simulink model "RP20231104WLR_231105"  (R2018b)
settings: Solver=FixedStepDiscrete  StartTime=0.0  StopTime=10.0  FixedStep=0.0005  RelTol=1e-3  EnableMultiTasking=on
undefined symbols (not defined in the file or in its folder): I_AN06_5V, I_AN07_5V, I_AN08_5V, I_AN09_5V, I_HALL1, I_SW01_L, O_SW12_HS1A, O_SW14_HS1A, PWM3
libraries: ec5744lib x60, simulink x33, canmsglib x5
(part 1 of 2)
settings Model: Creator=evil  LastModifiedBy=evil
settings SolverCC: AutoInsertRateTranBlk=on
settings OptimizationCC: DefaultParameterBehavior=Inlined  InlineInvariantSignals=on  EnhancedBackFolding=on  ExpressionFolding=off  PassReuseOutputArgsAs=Individual arguments  RollThreshold=65  StateBitsets=on  DataBitsets=on  ZeroExternalMemoryAtStartup=off  ZeroInternalMemoryAtStartup=off  EfficientFloat2IntCast=on  OptimizeBlockOrder=speed  DifferentSizesBufferReuse=on
settings DebuggingCC: InheritedTsInSrcMsg=none  ParameterTunabilityLossMsg=error
settings HardwareCC: ProdBitPerPointer=32  ProdBitPerSizeT=32  ProdBitPerPtrDiffT=32  ProdLargestAtomicInteger=Long  ProdLargestAtomicFloat=Double  ProdEndianess=BigEndian  ProdWordSize=32  ProdHWDeviceType=Freescale MPC5500
settings SFSimCC: MATLABDynamicMemAlloc=off
settings RTWCC: SystemTargetFile=ec5744.tlc  MakeCommand=make_rtw optimized_fixed_point=1  GenerateMakefile=off  TemplateMakefile=ec5744_lcc.tmf  PostCodeGenCommand=ec5744_pst_s2(buildInfo)  Description=Target for EC5744  GenerateReport=on  IncludeHyperlinkInReport=on  LaunchReport=on  GenerateTraceInfo=on  GenerateTraceReport=on  GenerateTraceReportSl=on  GenerateTraceReportSf=on  GenerateTraceReportEml=on
settings CodeAppCC: ForceParamTrailComments=on  IgnoreCustomStorageClasses=off  OperatorAnnotations=on  SimulinkDataObjDesc=on  SFDataObjDesc=on  InsertBlockDesc=on
settings STFCustomTargetCC: TargetLangStandard=C99 (ISO)  MultiwordLength=256  ModelReferenceCompliant=off  IncludeMdlTerminateFcn=off  CombineOutputUpdateFcns=on  SuppressErrorStatus=on  ERTCustomFileBanners=on  SupportContinuousTime=off  SupportNonInlinedSFcns=off  RemoveResetFunc=on  MATLABClassNameForMDSCustomization=Simulink.SoftwareTarget.ERTCustomization  SystemTargetFile=ec5744.tlc
settings ERTTargetCC: TargetLangStandard=C99 (ISO)  ModelReferenceCompliant=off  ParMdlRefBuildCompliant=off  CompOptLevelCompliant=off  ConcurrentExecutionCompliant=off  IncludeMdlTerminateFcn=off  SuppressErrorStatus=on  ModelStepFunctionPrototypeControlCompliant=off  CPPClassGenCompliant=off  UseToolchainInfoCompliant=off  GenerateASAP2=on  InlinedParameterPlacement=NonHierarchical  ERTSrcFileBannerTemplate=ec5744_code_template.cgt  ERTHdrFileBannerTemplate=ec5744_code_template.cgt  ERTDataSrcFileTemplate=ec5744_code_template.cgt  ERTDataHdrFileTemplate=ec5744_code_template.cgt  ERTCustomFileTemplate=ec5744_file_process.tlc

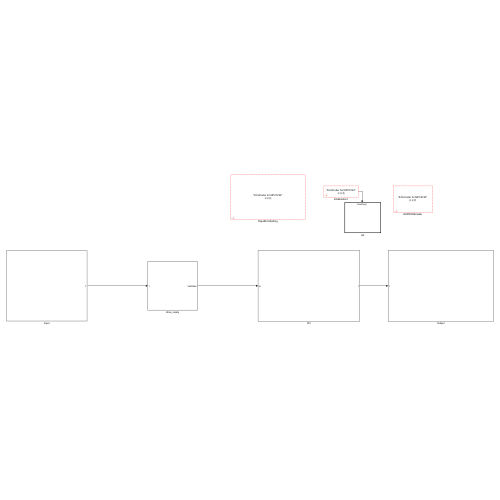
[thumbnail: Simulink's stored preview of the top-level diagram]
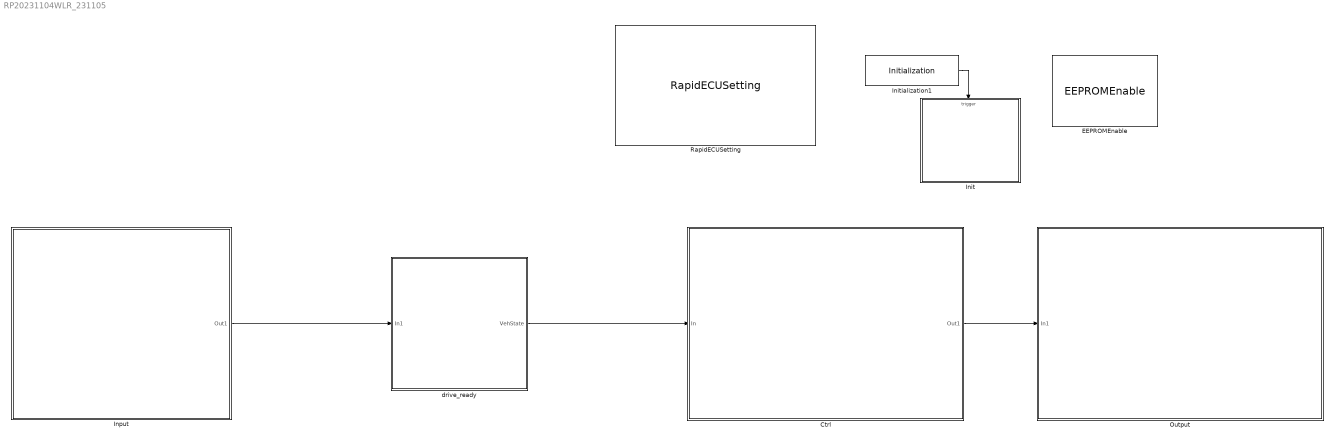
== system RP20231104WLR_231105 ==
  Ctrl : Subsystem
  EEPROMEnable : ec5744lib/RapidECU_U3/09MemoryManagement/EEPROMEnable  eepromenable=on
      settings: SourceProductName=ECUCoder for MPC5744
  Init : Subsystem  TreatAsAtomicUnit=on
  Initialization1 : ec5744lib/RapidECU_U3/08MCUManagement/Initialization
      settings: SourceProductName=ECUCoder for MPC5744
  Input : Subsystem
  Output : Subsystem
  RapidECUSetting : ec5744lib/RapidECU_U3/RapidECUSetting
      link override CAN: apdf=9  bpdf=4  cpdf=4  acmt=Extended(29-bit ID)  bcmt=Standard(11-bit ID)  ccmt=Standard(11-bit ID)
      link override LIN: abrt=19200
      settings: SourceProductName=ECUCoder for MPC5744
  drive_ready : Subsystem
  wires:
  Ctrl/1(Out1) -> Output/1(In1)
  Initialization1/1 -> Init/Trigger
  Input/1(Out1) -> drive_ready/1(In1)
  drive_ready/1(VehState) -> Ctrl/1(In)

== system RP20231104WLR_231105/Ctrl ==
  In : Inport
  10ms1 : simulink/Ports & Subsystems/Function-Call Generator  sample_time=0.01  numberOfIterations=1
  10ms5 : simulink/Ports & Subsystems/Function-Call Generator  sample_time=0.01  numberOfIterations=1
  Bus Creator1 : BusCreator  Inputs=3
  FAN_WP_CTRL : Subsystem  TreatAsAtomicUnit=on
  MoTrqReq : Subsystem  TreatAsAtomicUnit=on
  Out1 : Outport  VectorParamsAs1DForOutWhenUnconnected=on
  wires:
  10ms1/1 -> MoTrqReq/Trigger
  In/1 -> FAN_WP_CTRL/1(In), Bus Creator1/3, MoTrqReq/1(In)
  10ms5/1 -> FAN_WP_CTRL/Trigger
  MoTrqReq/1(Motor_CtrlBus) -> Bus Creator1/1  "Motor_CtrlBus"
  FAN_WP_CTRL/1(WP_FAN) -> Bus Creator1/2  "WP_FAN"
  Bus Creator1/1 -> Out1/1

== system RP20231104WLR_231105/Init ==
  function : TriggerPort  TriggerType=function-call  VariantControl=(inherit)
  AfterRunSwitch1 : ec5744lib/RapidECU_U3/05PowerManagement/AfterRunSwitch  sampletime=-1
      settings: SourceProductName=ECUCoder for MPC5744
  Constant : Constant  OutDataTypeStr=boolean
  Data Type Conversion : DataTypeConversion  OutDataTypeStr=boolean
  wires:
  Constant/1 -> Data Type Conversion/1
  Data Type Conversion/1 -> AfterRunSwitch1/1

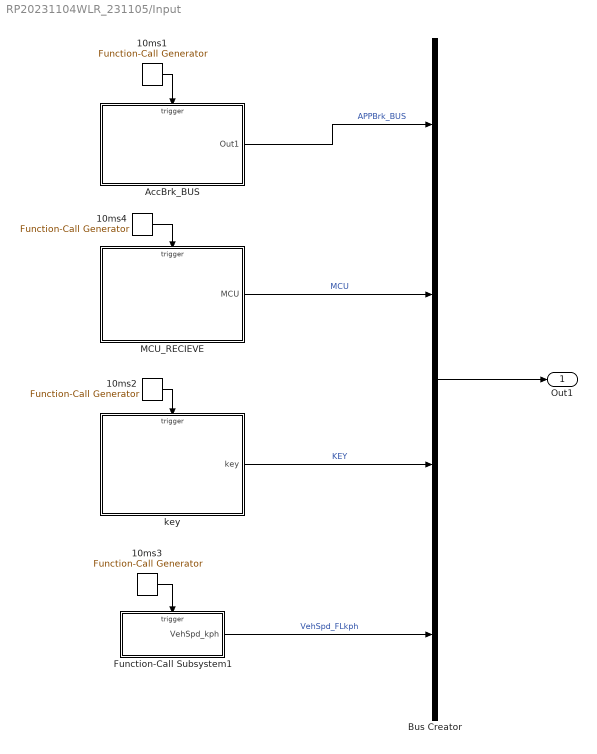
== system RP20231104WLR_231105/Input ==
  10ms{1..4} (4 alike) : simulink/Ports & Subsystems/Function-Call Generator  sample_time=0.01  numberOfIterations=1
  AccBrk_BUS : Subsystem  TreatAsAtomicUnit=on
  Bus Creator : BusCreator  Inputs=4
  Function-Call Subsystem1 : Subsystem  TreatAsAtomicUnit=on
  MCU_RECIEVE : Subsystem  TreatAsAtomicUnit=on
  key : Subsystem  TreatAsAtomicUnit=on
  Out1 : Outport  VectorParamsAs1DForOutWhenUnconnected=on
  wires:
  10ms1/1 -> AccBrk_BUS/Trigger
  MCU_RECIEVE/1(MCU) -> Bus Creator/2  "MCU"
  10ms4/1 -> MCU_RECIEVE/Trigger
  key/1(key) -> Bus Creator/3  "KEY"
  10ms2/1 -> key/Trigger
  Bus Creator/1 -> Out1/1
  AccBrk_BUS/1(Out1) -> Bus Creator/1  "APPBrk_BUS"
  10ms3/1 -> Function-Call Subsystem1/Trigger
  Function-Call Subsystem1/1(VehSpd_kph) -> Bus Creator/4  "VehSpd_FLkph"

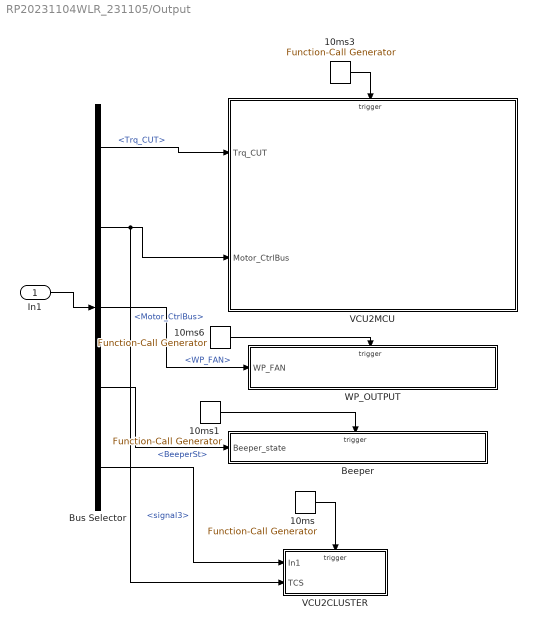
== system RP20231104WLR_231105/Output ==
  In1 : Inport
  10ms{,1,3,6} (4 alike) : simulink/Ports & Subsystems/Function-Call Generator  sample_time=0.01  numberOfIterations=1
  Beeper : Subsystem  TreatAsAtomicUnit=on
  Bus Selector : BusSelector  OutputSignals=signal3.signal2.APPBrk_BUS.Trq_CUT,Motor_CtrlBus,WP_FAN,signal3.VehState.BeeperSt,signal3
  VCU2CLUSTER : Subsystem  TreatAsAtomicUnit=on
  VCU2MCU : Subsystem  TreatAsAtomicUnit=on
  WP_OUTPUT : Subsystem  TreatAsAtomicUnit=on
  wires:
  10ms3/1 -> VCU2MCU/Trigger
  10ms6/1 -> WP_OUTPUT/Trigger
  In1/1 -> Bus Selector/1
  Bus Selector/1 -> VCU2MCU/1(Trq_CUT)  "<Trq_CUT>"
  Bus Selector/3 -> WP_OUTPUT/1(WP_FAN)  "<WP_FAN>"
  Bus Selector/2 -> VCU2CLUSTER/2(TCS), VCU2MCU/2(Motor_CtrlBus)  "<Motor_CtrlBus>"
  Bus Selector/4 -> Beeper/1(Beeper_state)  "<BeeperSt>"
  10ms1/1 -> Beeper/Trigger
  10ms/1 -> VCU2CLUSTER/Trigger
  Bus Selector/5 -> VCU2CLUSTER/1(In1)  "<signal3>"

== system RP20231104WLR_231105/drive_ready ==
  In1 : Inport
  10ms7 : simulink/Ports & Subsystems/Function-Call Generator  sample_time=0.01  numberOfIterations=1
  Bus Creator : BusCreator  Inputs=2
  Drive_ready : Subsystem  TreatAsAtomicUnit=on
  VehState : Outport
  wires:
  10ms7/1 -> Drive_ready/Trigger
  Drive_ready/1(VehStateBus) -> Bus Creator/1  "VehState"
  Bus Creator/1 -> VehState/1
  In1/1 -> Bus Creator/2, Drive_ready/1(BusIn)

== system RP20231104WLR_231105/Ctrl/FAN_WP_CTRL ==
  note: 1.温升做一个微分，根据温升速度来确定转速（温升系数）做到二维查表
      | 2.冷却要尽量做到刚刚好不过量，作热仿真（b站simulink热仿真）
  In : Inport
  function : TriggerPort  TriggerType=function-call  VariantControl=(inherit)
  Bus Creator : BusCreator  Inputs=1
  Bus Selector3 : BusSelector  OutputSignals=signal2.MCU.MCU_pwr.MCU_temp,signal2.MCU.MCU_pwr.motor_temp
  Data Type Conversion3 : DataTypeConversion  OutDataTypeStr=uint16
  Gain : Gain  Gain=10000/2000
  MCU__spd : Lookup_n-D  NumberOfTableDimensions=1  BreakpointsForDimension1=uint16([10,15,20,25,30,35,40,45,50,55,60,65,70,75]);  Table=uint16([0,0,600,600,600,600,800,800,800,1000,1000,1000,1000,1000]);  ExtrapMethod=Clip  InternalRulePriority=Speed  RndMeth=Simplest  InputSameDT=on
  MinMax : MinMax  Function=max  Inputs=2  OutDataTypeStr=uint16
  moter__spd : Lookup_n-D  NumberOfTableDimensions=1  BreakpointsForDimension1=uint16([0,10,20,30,40,50,60,70,80,90,100,110,120]);  Table=uint16([0,0,0,0,0,0,0,1400,1700,2000,2000,2000,2000]);  ExtrapMethod=Clip  InternalRulePriority=Speed  RndMeth=Simplest  InputSameDT=on
  WP_FAN : Outport  VectorParamsAs1DForOutWhenUnconnected=on
  wires:
  In/1 -> Bus Selector3/1
  Bus Selector3/1 -> MCU__spd/1  "<MCU_temp>"
  Bus Selector3/2 -> moter__spd/1  "<motor_temp>"
  MCU__spd/1 -> MinMax/1
  moter__spd/1 -> MinMax/2
  Bus Creator/1 -> WP_FAN/1
  MinMax/1 -> Gain/1  "Water_pump"
  Gain/1 -> Data Type Conversion3/1  "Water_pump"
  Data Type Conversion3/1 -> Bus Creator/1  "Water_pump"

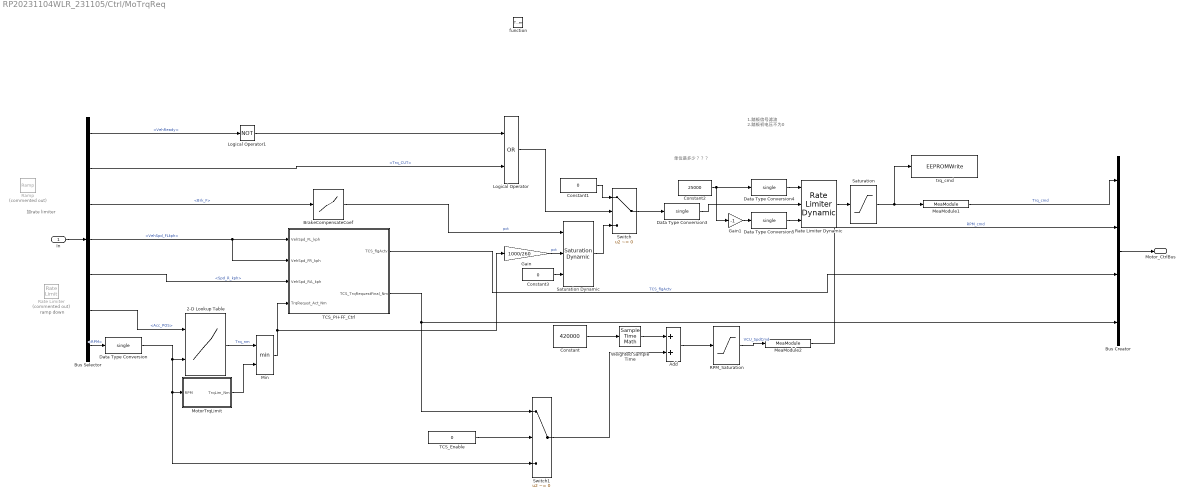
== system RP20231104WLR_231105/Ctrl/MoTrqReq ==
  note: 单位是多少？？？
  note: 加rate limiter
  note: ramp down
  note: 1.踏板信号滤波
      | 2.踏板初电压不为0
  In : Inport
  function : TriggerPort  TriggerType=function-call  VariantControl=(inherit)
  2-D Lookup Table : Lookup_n-D  BreakpointsForDimension1=single([0,10,20,30,40,50,60,70,80,90,100]);  BreakpointsForDimension2=single([200,400,600,800,1000,1200,1400,1600,1800,2000,2200,2400,2600,2800,3000,3500,4000,4500,5000,5200]);  BreakpointsForDimension1DataTypeStr=single  BreakpointsForDimension2DataTypeStr=single  Table=single(reshape([0,20,35,50,79,100,120,125,130,130,170,0,20,35,50,79,100,120,125,160,160,170,0,20,35,50,79,100,120,125,160,160,180,0,20,35,50,79,105,120,130,160,160,180,0,20,35,50,85,105,125,135,160,160,180,0,20,35,50,85,105,125,140,170,170,210,0,20,30,50,85,110,125,145,160,160,200,0,18,30,50,90,110,135,155,160,160,200,0,18,25,50,95,110,135,155,160,160,200,0,18,25,40,100,110,135,155,160,160,200,0,17,25,40,110,115,135,155,160,160,200,0,17,25,40,110,115,135,155,160,160,200,0,16,20,40,110,125,135,155,160,160,190,0,16,20,40,100,125,130,155,160,160,180,0,15,20,40,90,120,130,155,160,160,180,0,15,20,40,90,110,120,135,142,142,152,0,15,20,40,80,90,100,110,120,120,133,0,14,20,40,72,80,90,100,105,105,118,0,14,20,38,70,76,82,88,94,95,106,0,14,18,35,65,70,74,82,88,91,100],11,20));  InternalRulePriority=Speed  RndMeth=Simplest  InputSameDT=on
  Add : Sum
  BrakeCompensateCoef : Lookup_n-D  NumberOfTableDimensions=1  BreakpointsForDimension1=single([550,2000]);  Table=single([1000,0]);  ExtrapMethod=Clip  InternalRulePriority=Speed  OutDataTypeStr=single  RndMeth=Simplest  InputSameDT=on
  Bus Creator : BusCreator  Inputs=4
  Bus Selector : BusSelector  OutputSignals=VehState.VehReady,signal2.APPBrk_BUS.Trq_CUT,signal2.APPBrk_BUS.Brk_F,signal2.VehSpd_FLkph,signal2.MCU.MCU_state.Spd_R_kph,signal2.APPBrk_BUS.Acc_POS,signal2.MCU.MCU_state.RPM
  Constant : Constant  Value=420000  OutDataTypeStr=single
  Constant1 : Constant  Value=0  OutDataTypeStr=single
  Constant2 : Constant  Value=25000  OutDataTypeStr=single
  Constant3 : Constant  Value=0  OutDataTypeStr=single
  Data Type Conversion{,3..5} (4 alike) : DataTypeConversion  OutDataTypeStr=single
  Gain : Gain  Gain=1000/260
  Gain1 : Gain  Gain=-1
  Logical Operator : Logic  Operator=OR  AllPortsSameDT=off  OutDataTypeStr=boolean
  Logical Operator1 : Logic  Operator=NOT  AllPortsSameDT=off  OutDataTypeStr=boolean
  MeaModule1 : ec5744lib/HYFCU001/07Calibration/MeaModule  signal=VCU_TrqCmd
      settings: SourceProductName=ECUCoder for MPC5744
  MeaModule2 : ec5744lib/HYFCU001/07Calibration/MeaModule  signal=VCU_SpdCmd
      settings: SourceProductName=ECUCoder for MPC5744
  Min : MinMax  Inputs=2
  MotorTrqLimit : Subsystem
  RPM_Saturation : Saturate  UpperLimit=5000  LowerLimit=-50
  Ramp : simulink/Sources/Ramp  Commented=on  slope=1  start=0  InitialOutput=0
  Rate Limiter : RateLimiter  Commented=on  SampleTimeMode=inherited
  Rate Limiter Dynamic : simulink/Discontinuities/Rate Limiter Dynamic
  Saturation : Saturate  UpperLimit=1000  LowerLimit=-1000
  Saturation Dynamic : simulink/Discontinuities/Saturation Dynamic  OutMin=[]  OutMax=[]  OutDataTypeStr=single  OutputDataTypeScalingMode=single  OutDataType=fixdt(1, 16)  OutScaling=2^-10  DoSatur=off
  Switch : Switch  Criteria=u2 ~= 0
  Switch1 : Switch  Criteria=u2 ~= 0
  TCS_Enable : Constant  Value=0  OutDataTypeStr=boolean
  TCS_PI+FF_Ctrl : Subsystem
  Weighted Sample Time : SampleTimeMath  TsampMathOp=*
  trq_cmd : ec5744lib/RapidECU_U3/09MemoryManagement/EEPROMWrite  buffer=6  sampletime=-1
      settings: SourceProductName=ECUCoder for MPC5744
  Motor_CtrlBus : Outport
  wires:
  In/1 -> Bus Selector/1
  BrakeCompensateCoef/1 -> Saturation Dynamic/1  "pct"
  2-D Lookup Table/1 -> Min/1  "Trq_nm"
  Gain/1 -> Saturation Dynamic/2  "pct"
  Data Type Conversion/1 -> 2-D Lookup Table/2, Switch1/3, MotorTrqLimit/1(RPM)
  Rate Limiter Dynamic/1 -> Saturation/1
  Saturation/1 -> MeaModule1/1, trq_cmd/1
  Constant2/1 -> Data Type Conversion4/1, Gain1/1
  Data Type Conversion5/1 -> Rate Limiter Dynamic/3
  RPM_Saturation/1 -> MeaModule2/1  "VCU_SpdCmd"
  Data Type Conversion3/1 -> Rate Limiter Dynamic/2
  Data Type Conversion4/1 -> Rate Limiter Dynamic/1
  Gain1/1 -> Data Type Conversion5/1
  MeaModule2/1 -> Bus Creator/2  "RPM_cmd"
  Bus Creator/1 -> Motor_CtrlBus/1
  Add/1 -> RPM_Saturation/1
  Constant/1 -> Weighted Sample Time/1
  Weighted Sample Time/1 -> Add/1
  Switch/1 -> Data Type Conversion3/1
  Saturation Dynamic/1 -> Switch/3
  Constant1/1 -> Switch/1
  Bus Selector/7 -> Data Type Conversion/1  "<RPM>"
  Bus Selector/6 -> 2-D Lookup Table/1  "<Acc_POS>"
  Bus Selector/3 -> BrakeCompensateCoef/1  "<Brk_F>"
  Bus Selector/2 -> Logical Operator/2  "<Trq_CUT>"
  Logical Operator/1 -> Switch/2
  Bus Selector/1 -> Logical Operator1/1  "<VehReady>"
  Logical Operator1/1 -> Logical Operator/1
  MeaModule1/1 -> Bus Creator/1  "Trq_cmd"
  Constant3/1 -> Saturation Dynamic/3
  Bus Selector/4 -> TCS_PI+FF_Ctrl/2(VehSpd_FR_kph), TCS_PI+FF_Ctrl/1(VehSpd_FL_kph)  "<VehSpd_FLkph>"
  Bus Selector/5 -> TCS_PI+FF_Ctrl/3(VehSpd_RA_kph)  "<Spd_R_kph>"
  Min/1 -> TCS_PI+FF_Ctrl/4(TrqRequst_Act_Nm), Gain/1
  TCS_PI+FF_Ctrl/1(TCS_flgActv) -> Bus Creator/3  "TCS_flgActv"
  TCS_PI+FF_Ctrl/2(TCS_TrqRequestFinal_Nm) -> Bus Creator/4, Switch1/1
  MotorTrqLimit/1(TrqLim_Nm) -> Min/2
  TCS_Enable/1 -> Switch1/2
  Switch1/1 -> Add/2

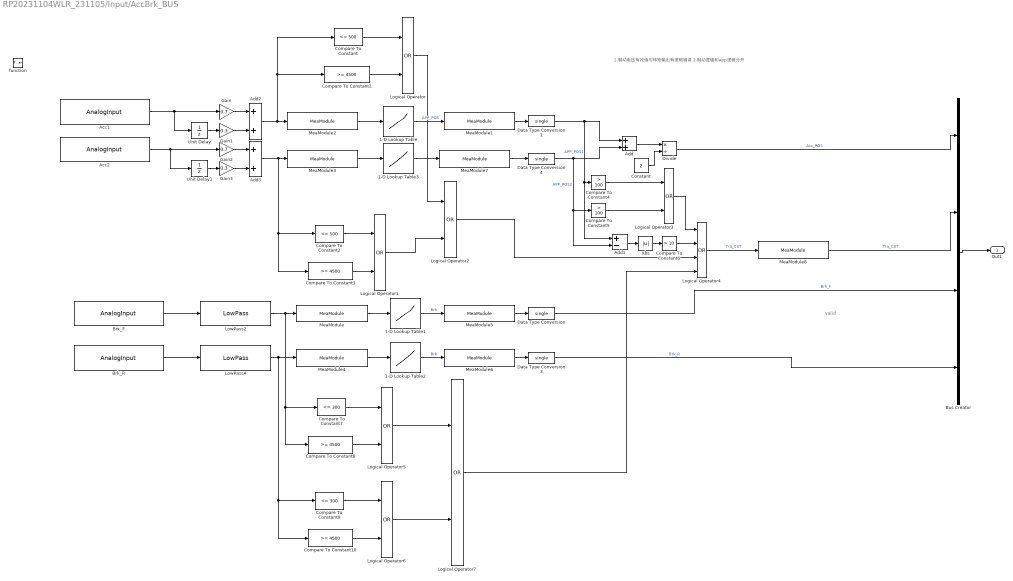
== system RP20231104WLR_231105/Input/AccBrk_BUS ==
  note: valid
  note: 1.制动电压有效值与转矩输出有逻辑错误
      | 2.制动逻辑和app逻辑分开
  function : TriggerPort  TriggerType=function-call  VariantControl=(inherit)
  1-D Lookup Table : Lookup_n-D  NumberOfTableDimensions=1  BreakpointsForDimension1=single([1330,1590]);  BreakpointsForDimension1DataTypeStr=single  Table=single([0,100]);  TableDataTypeStr=single  ExtrapMethod=Clip  InternalRulePriority=Speed  RndMeth=Simplest  InputSameDT=on
  1-D Lookup Table1 : Lookup_n-D  NumberOfTableDimensions=1  BreakpointsForDimension1=single([500,4500]);  BreakpointsForDimension1DataTypeStr=single  Table=single([0,10000]);  TableDataTypeStr=single  ExtrapMethod=Clip  InternalRulePriority=Speed  RndMeth=Simplest  InputSameDT=on
  1-D Lookup Table2 : Lookup_n-D  NumberOfTableDimensions=1  BreakpointsForDimension1=single([530,4500]);  BreakpointsForDimension1DataTypeStr=single  Table=single([0,10000]);  TableDataTypeStr=single  ExtrapMethod=Clip  InternalRulePriority=Speed  RndMeth=Simplest  InputSameDT=on
  1-D Lookup Table3 : Lookup_n-D  NumberOfTableDimensions=1  BreakpointsForDimension1=single([2324,2600]);  BreakpointsForDimension1DataTypeStr=single  Table=single([0,100]);  TableDataTypeStr=single  ExtrapMethod=Clip  InternalRulePriority=Speed  RndMeth=Simplest  InputSameDT=on
  Abs : Abs
  Acc1 : ec5744lib/RapidECU_U3/01BasicInput/AnalogInput  channel=52:I_AN06_5V  sampletime=-1
      settings: SourceProductName=ECUCoder for MPC5744
  Acc2 : ec5744lib/RapidECU_U3/01BasicInput/AnalogInput  channel=53:I_AN07_5V  sampletime=-1
      settings: SourceProductName=ECUCoder for MPC5744
  Add : Sum
  Add1 : Sum  Inputs=+-
  Add2 : Sum
  Add3 : Sum
  Brk_F : ec5744lib/RapidECU_U3/01BasicInput/AnalogInput  channel=54:I_AN08_5V  sampletime=-1
      settings: SourceProductName=ECUCoder for MPC5744
  Brk_R : ec5744lib/RapidECU_U3/01BasicInput/AnalogInput  channel=55:I_AN09_5V  sampletime=-1
      settings: SourceProductName=ECUCoder for MPC5744
  Bus Creator : BusCreator  Inputs=4
  Compare To Constant : simulink/Logic and Bit Operations/Compare To Constant  relop=<=  const=500  OutDataTypeStr=boolean
  Compare To Constant{1,3,8,10} (4 alike) : simulink/Logic and Bit Operations/Compare To Constant  relop=>=  const=4500  OutDataTypeStr=boolean
  Compare To Constant2 : simulink/Logic and Bit Operations/Compare To Constant  relop=<=  const=500  OutDataTypeStr=boolean
  Compare To Constant4 : simulink/Logic and Bit Operations/Compare To Constant  relop=>  const=100  OutDataTypeStr=boolean
  Compare To Constant5 : simulink/Logic and Bit Operations/Compare To Constant  relop=>  const=100  OutDataTypeStr=boolean
  Compare To Constant6 : simulink/Logic and Bit Operations/Compare To Constant  relop=>  const=10  OutDataTypeStr=boolean
  Compare To Constant7 : simulink/Logic and Bit Operations/Compare To Constant  relop=<=  const=300  OutDataTypeStr=boolean
  Compare To Constant9 : simulink/Logic and Bit Operations/Compare To Constant  relop=<=  const=300  OutDataTypeStr=boolean
  Constant : Constant  Value=2
  Data Type Conversion{,1,3..4} (4 alike) : DataTypeConversion  OutDataTypeStr=single
  Divide : Product  Inputs=*/  OutDataTypeStr=single
  Gain : Gain  Gain=0.7
  Gain1 : Gain  Gain=0.3
  Gain2 : Gain  Gain=0.7
  Gain3 : Gain  Gain=0.3
  Logical Operator{,1..3,5..7} (7 alike) : Logic  Operator=OR  AllPortsSameDT=off  OutDataTypeStr=boolean
  Logical Operator4 : Logic  Operator=OR  Inputs=4  AllPortsSameDT=off  OutDataTypeStr=boolean
  LowPass2 : ec5744lib/FrequentlyUsedModels/LowPass  coefficient=0.7
      settings: SourceProductName=ECUCoder for MPC5744
  LowPass4 : ec5744lib/FrequentlyUsedModels/LowPass  coefficient=0.7
      settings: SourceProductName=ECUCoder for MPC5744
  MeaModule : ec5744lib/RapidECU_U3/07Calibration/MeaModule  signal=Brk_F_vol
      settings: SourceProductName=ECUCoder for MPC5744
  MeaModule1 : ec5744lib/RapidECU_U3/07Calibration/MeaModule  signal=Acc_POS1
      settings: SourceProductName=ECUCoder for MPC5744
  MeaModule2 : ec5744lib/RapidECU_U3/07Calibration/MeaModule  signal=Acc_vol
      settings: SourceProductName=ECUCoder for MPC5744
  MeaModule3 : ec5744lib/RapidECU_U3/07Calibration/MeaModule  signal=Acc_vol2
      settings: SourceProductName=ECUCoder for MPC5744
  MeaModule4 : ec5744lib/RapidECU_U3/07Calibration/MeaModule  signal=Brk_R_vol
      settings: SourceProductName=ECUCoder for MPC5744
  MeaModule5 : ec5744lib/RapidECU_U3/07Calibration/MeaModule  signal=F_BrkPrs
      settings: SourceProductName=ECUCoder for MPC5744
  MeaModule6 : ec5744lib/RapidECU_U3/07Calibration/MeaModule  signal=R_BrkPrs
      settings: SourceProductName=ECUCoder for MPC5744
  MeaModule7 : ec5744lib/RapidECU_U3/07Calibration/MeaModule  signal=Acc_POS2
      settings: SourceProductName=ECUCoder for MPC5744
  MeaModule8 : ec5744lib/RapidECU_U3/07Calibration/MeaModule  signal=Trq_CUT
      settings: SourceProductName=ECUCoder for MPC5744
  Unit Delay : UnitDelay  SampleTime=-1
  Unit Delay1 : UnitDelay  SampleTime=-1
  Out1 : Outport
  wires:
  Bus Creator/1 -> Out1/1
  1-D Lookup Table/1 -> MeaModule1/1  "APP_POS"
  Acc1/1 -> Gain/1, Unit Delay/1
  MeaModule/1 -> 1-D Lookup Table1/1
  MeaModule1/1 -> Data Type Conversion1/1
  MeaModule2/1 -> 1-D Lookup Table/1
  Brk_F/1 -> LowPass2/1
  1-D Lookup Table1/1 -> MeaModule5/1  "Brk"
  MeaModule3/1 -> 1-D Lookup Table3/1
  1-D Lookup Table3/1 -> MeaModule7/1
  Brk_R/1 -> LowPass4/1
  1-D Lookup Table2/1 -> MeaModule6/1  "Brk"
  MeaModule4/1 -> 1-D Lookup Table2/1
  MeaModule5/1 -> Data Type Conversion/1
  MeaModule6/1 -> Data Type Conversion3/1
  MeaModule7/1 -> Data Type Conversion4/1
  Data Type Conversion1/1 -> Add1/1, Compare To Constant4/1, Add/1  "APP_POS1"
  Data Type Conversion4/1 -> Add1/2, Compare To Constant5/1, Add/2  "APP_POS2"
  Add/1 -> Divide/1
  Constant/1 -> Divide/2
  Divide/1 -> Bus Creator/1  "Acc_POS"
  Compare To Constant1/1 -> Logical Operator/2
  Compare To Constant/1 -> Logical Operator/1
  Add2/1 -> Compare To Constant/1, Compare To Constant1/1, MeaModule2/1
  Logical Operator/1 -> Logical Operator2/1
  Compare To Constant3/1 -> Logical Operator1/2
  Compare To Constant2/1 -> Logical Operator1/1
  Add3/1 -> Compare To Constant3/1, Compare To Constant2/1, MeaModule3/1
  Logical Operator1/1 -> Logical Operator2/2
  Compare To Constant4/1 -> Logical Operator3/1
  Compare To Constant5/1 -> Logical Operator3/2
  Logical Operator3/1 -> Logical Operator4/1
  Add1/1 -> Abs/1
  Abs/1 -> Compare To Constant6/1
  Compare To Constant6/1 -> Logical Operator4/2
  Logical Operator2/1 -> Logical Operator4/3
  Logical Operator4/1 -> MeaModule8/1  "Trq_CUT"
  Compare To Constant7/1 -> Logical Operator5/1
  Compare To Constant8/1 -> Logical Operator5/2
  LowPass2/1 -> Compare To Constant8/1, Compare To Constant7/1, MeaModule/1
  Logical Operator5/1 -> Logical Operator7/1
  Compare To Constant9/1 -> Logical Operator6/1
  Compare To Constant10/1 -> Logical Operator6/2
  LowPass4/1 -> Compare To Constant10/1, Compare To Constant9/1, MeaModule4/1
  Logical Operator6/1 -> Logical Operator7/2
  Logical Operator7/1 -> Logical Operator4/4
  Data Type Conversion/1 -> Bus Creator/3  "Brk_F"
  Data Type Conversion3/1 -> Bus Creator/4  "Brk_R"
  MeaModule8/1 -> Bus Creator/2  "Trq_CUT"
  Gain/1 -> Add2/1
  Unit Delay/1 -> Gain1/1
  Gain1/1 -> Add2/2
  Gain3/1 -> Add3/2
  Unit Delay1/1 -> Gain3/1
  Gain2/1 -> Add3/1
  Acc2/1 -> Unit Delay1/1, Gain2/1

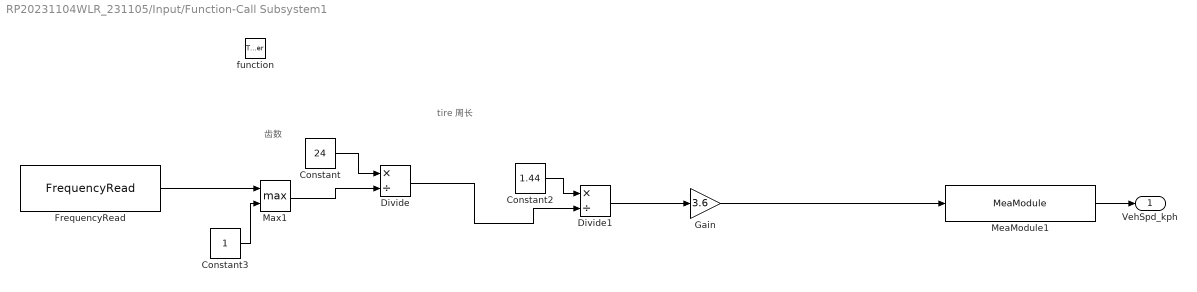
== system RP20231104WLR_231105/Input/Function-Call Subsystem1 ==
  note: 齿数
  note: tire 周长
  function : TriggerPort  TriggerType=function-call  VariantControl=Variant
  Constant : Constant  Value=24
  Constant2 : Constant  Value=1.44
  Constant3 : Constant
  Divide : Product  Inputs=*/
  Divide1 : Product  Inputs=*/
  FrequencyRead : ec5744lib/RapidECU_U3/01BasicInput/FrequencyRead  channel=37:I_HALL1  sampletime=-1
      settings: SourceProductName=ECUCoder for MPC5744
  Gain : Gain  Gain=3.6
  Max1 : MinMax  Function=max  Inputs=2
  MeaModule1 : ec5744lib/RapidECU_U3/07Calibration/MeaModule  signal=Wheel_spd_F
      settings: SourceProductName=ECUCoder for MPC5744
  VehSpd_kph : Outport
  wires:
  MeaModule1/1 -> VehSpd_kph/1
  Constant/1 -> Divide/1
  Divide/1 -> Divide1/2
  Constant2/1 -> Divide1/1
  Divide1/1 -> Gain/1
  Constant3/1 -> Max1/2
  FrequencyRead/1 -> Max1/1
  Max1/1 -> Divide/2
  Gain/1 -> MeaModule1/1

== system RP20231104WLR_231105/Input/MCU_RECIEVE ==
  function : TriggerPort  TriggerType=function-call  VariantControl=(inherit)
  Bus Creator2 : BusCreator  Inputs=2
  CANReceive1 : ec5744lib/RapidECU_U3/04CANCommunication/CANReceive  canmodule=0  canbuffer=1  canmessageid=218089455  canmessagetype=Extended(29-bit ID)  datalength=8  sampletime=-1
      settings: SourceProductName=ECUCoder for MPC5744
  CANReceive3 : ec5744lib/RapidECU_U3/04CANCommunication/CANReceive  canmodule=0  canbuffer=0  canmessageid=218089199  canmessagetype=Extended(29-bit ID)  datalength=8  sampletime=-1
      settings: SourceProductName=ECUCoder for MPC5744
  MCU_pwr : Subsystem  TreatAsAtomicUnit=on
  MCU_state : Subsystem  TreatAsAtomicUnit=on
  Terminator1 : Terminator
  Terminator3 : Terminator
  MCU : Outport  VectorParamsAs1DForOutWhenUnconnected=on
  wires:
  CANReceive1/3 -> MCU_pwr/2(ID)
  CANReceive1/4 -> MCU_pwr/3(Msg)
  CANReceive1/2 -> MCU_pwr/1(CANOK)
  CANReceive3/1 -> MCU_state/Trigger
  CANReceive1/1 -> MCU_pwr/Trigger
  MCU_pwr/1(MCU_pwr) -> Bus Creator2/2  "MCU_pwr"
  CANReceive3/2 -> MCU_state/1(CANOK)
  CANReceive3/5 -> Terminator3/1
  CANReceive1/5 -> Terminator1/1
  MCU_state/1(Out1) -> Bus Creator2/1  "MCU_state"
  CANReceive3/3 -> MCU_state/2(ID)
  CANReceive3/4 -> MCU_state/3(Msg)
  Bus Creator2/1 -> MCU/1

== system RP20231104WLR_231105/Input/key ==
  function : TriggerPort  TriggerType=function-call  VariantControl=(inherit)
  Bus Creator : BusCreator  Inputs=2
  KL15Monitor : ec5744lib/RapidECU_U3/05PowerManagement/KL15Monitor  sampletime=-1
      settings: SourceProductName=ECUCoder for MPC5744
  Logical Operator : Logic  Operator=NOT  AllPortsSameDT=off  OutDataTypeStr=boolean
  MeaModule : ec5744lib/RapidECU_U3/07Calibration/MeaModule  signal=ignition
      settings: SourceProductName=ECUCoder for MPC5744
  SwitchInput : ec5744lib/RapidECU_U3/01BasicInput/SwitchInput  channel=6:I_SW01_L  sampletime=-1
      settings: SourceProductName=ECUCoder for MPC5744
  key : Outport
  wires:
  SwitchInput/1 -> Logical Operator/1  "Drive_ready"
  KL15Monitor/1 -> Bus Creator/1  "LVMS"
  Bus Creator/1 -> key/1
  MeaModule/1 -> Bus Creator/2  "ignition"
  Logical Operator/1 -> MeaModule/1

== system RP20231104WLR_231105/Output/Beeper ==
  Beeper_state : Inport
  function : TriggerPort  TriggerType=function-call  VariantControl=(inherit)
  MeaModule : ec5744lib/RapidECU_U3/07Calibration/MeaModule  signal=beeper_state
      settings: SourceProductName=ECUCoder for MPC5744
  PowerDriverSwitch(HS) : ec5744lib/RapidECU_U3/02PowerDriverSwitch/PowerDriverSwitch(HS)  channel=117:O_SW14_HS1A  sampletime=-1
      settings: SourceProductName=ECUCoder for MPC5744
  wires:
  Beeper_state/1 -> MeaModule/1
  MeaModule/1 -> PowerDriverSwitch(HS)/1

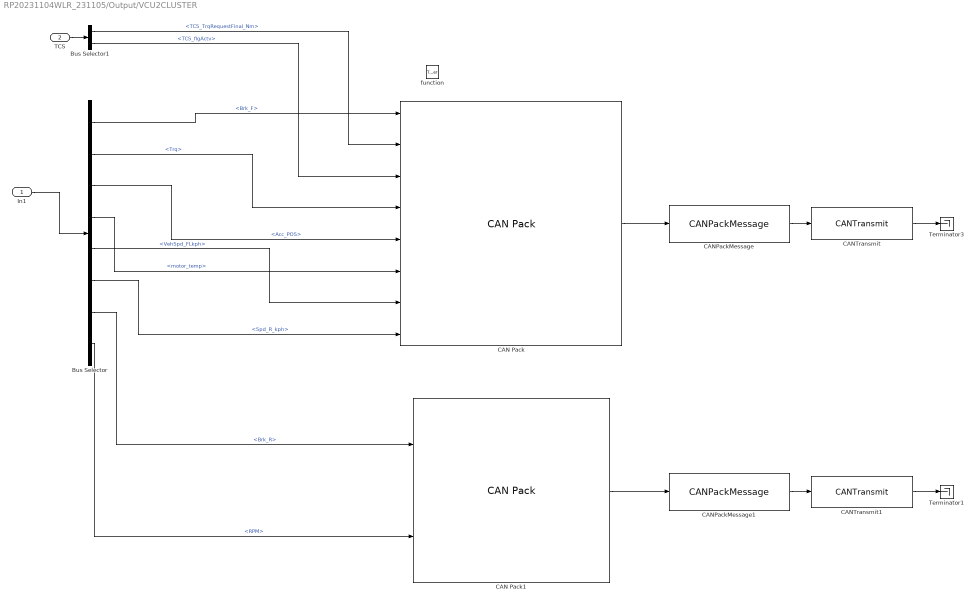
== system RP20231104WLR_231105/Output/VCU2CLUSTER ==
  In1 : Inport
  TCS : Inport  Port=2
  function : TriggerPort  TriggerType=function-call  VariantControl=Variant
  Bus Selector : BusSelector  OutputSignals=signal2.APPBrk_BUS.Brk_F,signal2.MCU.MCU_state.Trq,signal2.APPBrk_BUS.Acc_POS,signal2.MCU.MCU_pwr.motor_temp,signal2.VehSpd_FLkph,signal2.MCU.MCU_state.Spd_R_kph,signal2.APPBrk_BUS.Brk_R,signal2.MCU.MCU_state.RPM
  Bus Selector1 : BusSelector  OutputSignals=TCS_TrqRequestFinal_Nm,TCS_flgActv
  CAN Pack : canmsglib/CAN Pack  CANdbFile=E:\candbc\cluster.dbc  MsgList=New_Message_1  MsgName=New_Message_1  MsgIDType=Standard (11-bit identifier)  MsgIdentifier=291  MsgLength=8  SignalInfo=Brk_F$56$8$1$1$1$0$30$100$-3740$3910$#TCS_Trq_cmd$40$8$1$2$1$0$1$0$0$255$#TCS_flag$32$8$1$1$1$0$1$0$-Inf$Inf$#Trq_feedback$48$8$1$1$1$0$1$0$-128$250$#acc$24$8$1$2$1$0$1$0$0$100$#motor_temp$0$8$1$2$1$0$1$0$0$100$#veh_spd_F$8$8$1$2$1$0$1$0$0$120$#veh_spd_R$16$8$1$2$1$0$1$0$0$120$#  NSignals=8  StartBits=str2num('[int32(56);int32(40);int32(32);int32(48);int32(24);int32(0);int32(8);int32(16)]')  SignalSizes=str2num('[int32(8);int32(8);int32(8);int32(8);int32(8);int32(8);int32(8);int32(8)]')  ByteOrders=str2num('[int32(1);int32(1);int32(1);int32(1);int32(1);int32(1);int32(1);int32(1)]')  DataTypes=str2num('[int32(1);int32(2);int32(1);int32(1);int32(2);int32(2);int32(2);int32(2)]')  MultiplexTypes=str2num('[int32(1);int32(1);int32(1);int32(1);int32(1);int32(1);int32(1);int32(1)]')  MultiplexValues=str2num('[double(0);double(0);double(0);double(0);double(0);double(0);double(0);double(0)]')  Factors=str2num('[double(30);double(1);double(1);double(1);double(1);double(1);double(1);double(1)]')  Offsets=str2num('[double(100);double(0);double(0);double(0);double(0);double(0);double(0);double(0)]')  Minimums=str2num('[double(-3740);double(0);double(-Inf);double(-128);double(0);double(0);double(0);double(0)]')  Maximums=str2num('[double(3910);double(255);double(Inf);double(250);double(100);double(100);double(120);double(120)]')  Remote=off  ApplyMinMax=off  BusOutput=off
      settings: SourceProductBaseCode=XP,ME,VN  DataFormat=CANdb specified signals
  CAN Pack1 : canmsglib/CAN Pack  CANdbFile=E:\candbc\cluster.dbc  MsgList=New_Message_2  MsgName=New_Message_2  MsgIDType=Standard (11-bit identifier)  MsgIdentifier=292  MsgLength=2  SignalInfo=Brk_R$0$8$1$1$1$0$30$100$-Inf$Inf$#RPM_feedback$8$8$1$1$1$0$1$0$-Inf$Inf$#  NSignals=2  StartBits=str2num('[int32(0);int32(8)]')  SignalSizes=str2num('[int32(8);int32(8)]')  ByteOrders=str2num('[int32(1);int32(1)]')  DataTypes=str2num('[int32(1);int32(1)]')  MultiplexTypes=str2num('[int32(1);int32(1)]')  MultiplexValues=str2num('[double(0);double(0)]')  Factors=str2num('[double(30);double(1)]')  Offsets=str2num('[double(100);double(0)]')  Minimums=str2num('[double(-Inf);double(-Inf)]')  Maximums=str2num('[double(Inf);double(Inf)]')  Remote=off  ApplyMinMax=off  BusOutput=off
      settings: SourceProductName=Simulink Real-Time  SourceProductBaseCode=XP  DataFormat=CANdb specified signals
  CANPackMessage : ec5744lib/RapidECU_U3/04CANCommunication/CANPackMessage  datalength=8  sampletime=-1
      settings: SourceProductName=ECUCoder for MPC5744
  CANPackMessage1 : ec5744lib/HYFCU001/04CANCommunication/CANPackMessage  datalength=8  sampletime=-1
      settings: SourceProductName=ECUCoder for MPC5744
  CANTransmit : ec5744lib/RapidECU_U3/04CANCommunication/CANTransmit  canmodule=0  canbuffer=9  canmessageid=291  canmessagetype=Standard(11-bit ID)  datalength=8  sampletime=-1
      settings: SourceProductName=ECUCoder for MPC5744
  CANTransmit1 : ec5744lib/RapidECU_U3/04CANCommunication/CANTransmit  canmodule=0  canbuffer=10  canmessageid=292  canmessagetype=Standard(11-bit ID)  datalength=8  sampletime=-1
      settings: SourceProductName=ECUCoder for MPC5744
  Terminator1 : Terminator
  Terminator3 : Terminator
  wires:
  CANTransmit/1 -> Terminator3/1
  CANPackMessage/1 -> CANTransmit/1
  CAN Pack/1 -> CANPackMessage/1
  In1/1 -> Bus Selector/1
  Bus Selector/5 -> CAN Pack/7  "<VehSpd_FLkph>"
  Bus Selector/4 -> CAN Pack/6  "<motor_temp>"
  Bus Selector/3 -> CAN Pack/5  "<Acc_POS>"
  Bus Selector/6 -> CAN Pack/8  "<Spd_R_kph>"
  Bus Selector/1 -> CAN Pack/1  "<Brk_F>"
  Bus Selector/2 -> CAN Pack/4  "<Trq>"
  TCS/1 -> Bus Selector1/1
  Bus Selector1/2 -> CAN Pack/3  "<TCS_flgActv>"
  Bus Selector1/1 -> CAN Pack/2  "<TCS_TrqRequestFinal_Nm>"
  Bus Selector/7 -> CAN Pack1/1  "<Brk_R>"
  Bus Selector/8 -> CAN Pack1/2  "<RPM>"
  CAN Pack1/1 -> CANPackMessage1/1
  CANPackMessage1/1 -> CANTransmit1/1
  CANTransmit1/1 -> Terminator1/1

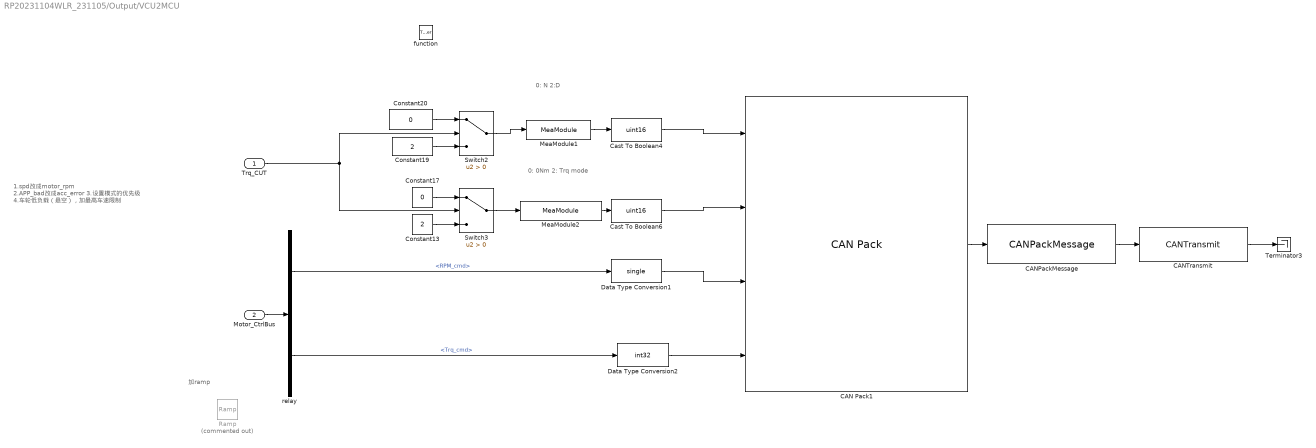
== system RP20231104WLR_231105/Output/VCU2MCU ==
  note: 0: 0Nm
      | 2: Trq mode
  note: 0: N
      | 2:D
  note: 加ramp
  note: 1.spd改成motor_rpm
      | 2.APP_bad改成acc_error
      | 3.设置模式的优先级
      | 4.车轮低负载（悬空），加最高车速限制
  Trq_CUT : Inport
  Motor_CtrlBus : Inport  Port=2
  function : TriggerPort  TriggerType=function-call  VariantControl=(inherit)
  CAN Pack1 : canmsglib/CAN Pack  CANdbFile=E:\candbc\MCU_No1.dbc  MsgList=(none)  MsgName=VCU2MCU1_ID1  MsgIDType=Extended (29-bit identifier)  MsgIdentifier=146927393  MsgLength=8  SignalInfo=VCU2MCU_Control_mode_ID1$32$8$1$2$1$0$1$0$0$255$#VCU2MCU_Gear_ID1$40$2$1$2$1$0$1$0$0$3$#VCU2MCU_Speed_Limit_ID1$0$16$1$2$1$0$5.000000e-01$-10000$-10000$10000$#VCU2MCU_Torque_Control_ID1$16$16$1$2$1$0$1$0$0$1000$#  NSignals=4  StartBits=str2num('[int32(32);int32(40);int32(0);int32(16)]')  SignalSizes=str2num('[int32(8);int32(2);int32(16);int32(16)]')  ByteOrders=str2num('[int32(1);int32(1);int32(1);int32(1)]')  DataTypes=str2num('[int32(2);int32(2);int32(2);int32(2)]')  MultiplexTypes=str2num('[int32(1);int32(1);int32(1);int32(1)]')  MultiplexValues=str2num('[double(0);double(0);double(0);double(0)]')  Factors=str2num('[double(1);double(1);double(5.000000e-01);double(1)]')  Offsets=str2num('[double(0);double(0);double(-10000);double(0)]')  Minimums=str2num('[double(0);double(0);double(-10000);double(0)]')  Maximums=str2num('[double(255);double(3);double(10000);double(1000)]')  Remote=off  ApplyMinMax=off  BusOutput=off
      settings: SourceProductBaseCode=XP,ME,VN  DataFormat=CANdb specified signals
  CANPackMessage : ec5744lib/RapidECU_U3/04CANCommunication/CANPackMessage  datalength=8  sampletime=-1
      settings: SourceProductName=ECUCoder for MPC5744
  CANTransmit : ec5744lib/RapidECU_U3/04CANCommunication/CANTransmit  canmodule=0  canbuffer=8  canmessageid=146927393  canmessagetype=Extended(29-bit ID)  datalength=8  sampletime=-1
      settings: SourceProductName=ECUCoder for MPC5744
  Cast To Boolean4 : DataTypeConversion  OutDataTypeStr=uint16
  Cast To Boolean6 : DataTypeConversion  OutDataTypeStr=uint16
  Constant13 : Constant  Value=2
  Constant17 : Constant  Value=0
  Constant19 : Constant  Value=2
  Constant20 : Constant  Value=0
  Data Type Conversion1 : DataTypeConversion  OutDataTypeStr=single
  Data Type Conversion2 : DataTypeConversion  OutDataTypeStr=int32
  MeaModule1 : ec5744lib/HYFCU001/07Calibration/MeaModule  signal=Gear_Trs
      settings: SourceProductName=ECUCoder for MPC5744
  MeaModule2 : ec5744lib/HYFCU001/07Calibration/MeaModule  signal=Mode_Trs
      settings: SourceProductName=ECUCoder for MPC5744
  Ramp : simulink/Sources/Ramp  Commented=on  slope=1  start=0  InitialOutput=0
  Switch2 : Switch  Criteria=u2 > Threshold
  Switch3 : Switch  Criteria=u2 > Threshold
  Terminator3 : Terminator
  relay : BusSelector  OutputSignals=RPM_cmd,Trq_cmd
  wires:
  CANTransmit/1 -> Terminator3/1
  relay/1 -> Data Type Conversion1/1  "<RPM_cmd>"
  CAN Pack1/1 -> CANPackMessage/1
  CANPackMessage/1 -> CANTransmit/1
  Motor_CtrlBus/1 -> relay/1
  MeaModule1/1 -> Cast To Boolean4/1
  relay/2 -> Data Type Conversion2/1  "<Trq_cmd>"
  Constant20/1 -> Switch2/1
  Trq_CUT/1 -> Switch2/2, Switch3/2
  Constant19/1 -> Switch2/3
  Constant13/1 -> Switch3/3
  Constant17/1 -> Switch3/1
  Switch3/1 -> MeaModule2/1
  Switch2/1 -> MeaModule1/1
  MeaModule2/1 -> Cast To Boolean6/1
  Data Type Conversion1/1 -> CAN Pack1/3
  Data Type Conversion2/1 -> CAN Pack1/4
  Cast To Boolean4/1 -> CAN Pack1/1
  Cast To Boolean6/1 -> CAN Pack1/2

== system RP20231104WLR_231105/Output/WP_OUTPUT ==
  note: 数据类型转换
  WP_FAN : Inport
  function : TriggerPort  TriggerType=function-call  VariantControl=(inherit)
  Bus Selector : BusSelector  OutputSignals=Water_pump
  Constant : Constant  Value=1000  OutDataTypeStr=uint16  SampleTime=-1
  PowerDriverPWM : ec5744lib/RapidECU_U3/03PowerDriverPWM/PowerDriverPWM  channel=114:O_SW12_HS1A/PWM3  sampletime=-1
      settings: SourceProductName=ECUCoder for MPC5744
  wires:
  Bus Selector/1 -> PowerDriverPWM/2  "<Water_pump>"
  Constant/1 -> PowerDriverPWM/1
  WP_FAN/1 -> Bus Selector/1

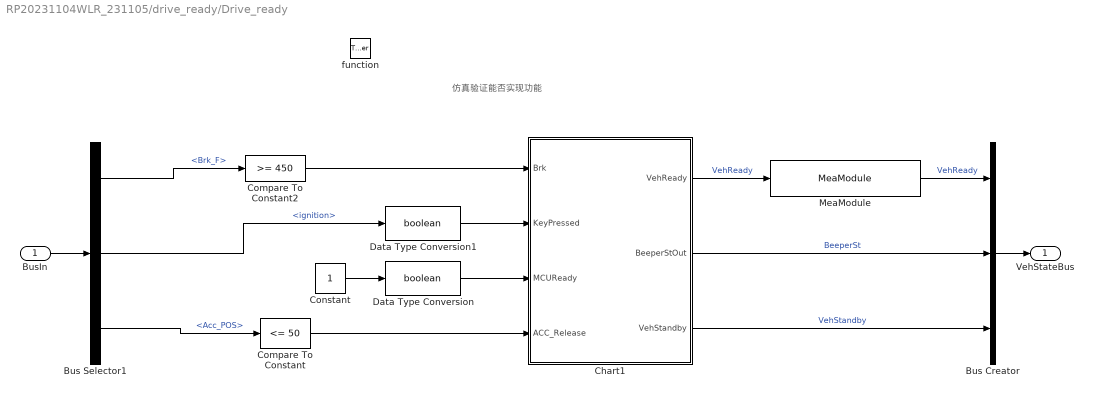
== system RP20231104WLR_231105/drive_ready/Drive_ready ==
  note: 仿真验证能否实现功能
  BusIn : Inport
  function : TriggerPort  TriggerType=function-call  VariantControl=(inherit)
  Bus Creator : BusCreator  Inputs=3
  Bus Selector1 : BusSelector  OutputSignals=APPBrk_BUS.Brk_F,KEY.ignition,APPBrk_BUS.Acc_POS
  Chart1 : Stateflow chart  TreatAsAtomicUnit=on
  Compare To Constant : simulink/Logic and Bit Operations/Compare To Constant  relop=<=  const=50  OutDataTypeStr=boolean
  Compare To Constant2 : simulink/Logic and Bit Operations/Compare To Constant  relop=>=  const=450  OutDataTypeStr=boolean
  Constant : Constant
  Data Type Conversion : DataTypeConversion  OutDataTypeStr=boolean  RndMeth=Nearest
  Data Type Conversion1 : DataTypeConversion  OutDataTypeStr=boolean  RndMeth=Nearest
  MeaModule : ec5744lib/RapidECU_U3/07Calibration/MeaModule  signal=VehReady
      settings: SourceProductName=ECUCoder for MPC5744
  VehStateBus : Outport
  wires:
  Bus Selector1/1 -> Compare To Constant2/1  "<Brk_F>"
  Bus Selector1/2 -> Data Type Conversion1/1  "<ignition>"
  BusIn/1 -> Bus Selector1/1
  Chart1/1(VehReady) -> MeaModule/1  "VehReady"
  Chart1/3(VehStandby) -> Bus Creator/3  "VehStandby"
  Compare To Constant2/1 -> Chart1/1(Brk)
  Bus Selector1/3 -> Compare To Constant/1  "<Acc_POS>"
  Compare To Constant/1 -> Chart1/4(ACC_Release)
  Data Type Conversion/1 -> Chart1/3(MCUReady)
  Data Type Conversion1/1 -> Chart1/2(KeyPressed)
  Chart1/2(BeeperStOut) -> Bus Creator/2  "BeeperSt"
  Bus Creator/1 -> VehStateBus/1
  MeaModule/1 -> Bus Creator/1  "VehReady"
  Constant/1 -> Data Type Conversion/1

== system RP20231104WLR_231105/Ctrl/MoTrqReq/MotorTrqLimit ==
  RPM : Inport
  Add1 : Sum
  Constant5 : Constant  Value=single(9550)  OutDataTypeStr=single
  Divide : Product  Inputs=*/
  Max : MinMax  Function=max  Inputs=2
  MaxPwr : Constant  Value=single(70)  OutDataTypeStr=single
  Product : Product
  RPM_min : Constant  Value=single(10)  OutDataTypeStr=single
  RPM_min1 : Constant  Value=single(1)  OutDataTypeStr=single
  TrqLim_Nm : Outport  VectorParamsAs1DForOutWhenUnconnected=on
  wires:
  Add1/1 -> Max/1
  MaxPwr/1 -> Product/1
  RPM_min/1 -> Add1/2
  RPM/1 -> Add1/1
  Product/1 -> Divide/1
  Constant5/1 -> Product/2
  Divide/1 -> TrqLim_Nm/1  "TrqLim_Nm"
  RPM_min1/1 -> Max/2
  Max/1 -> Divide/2

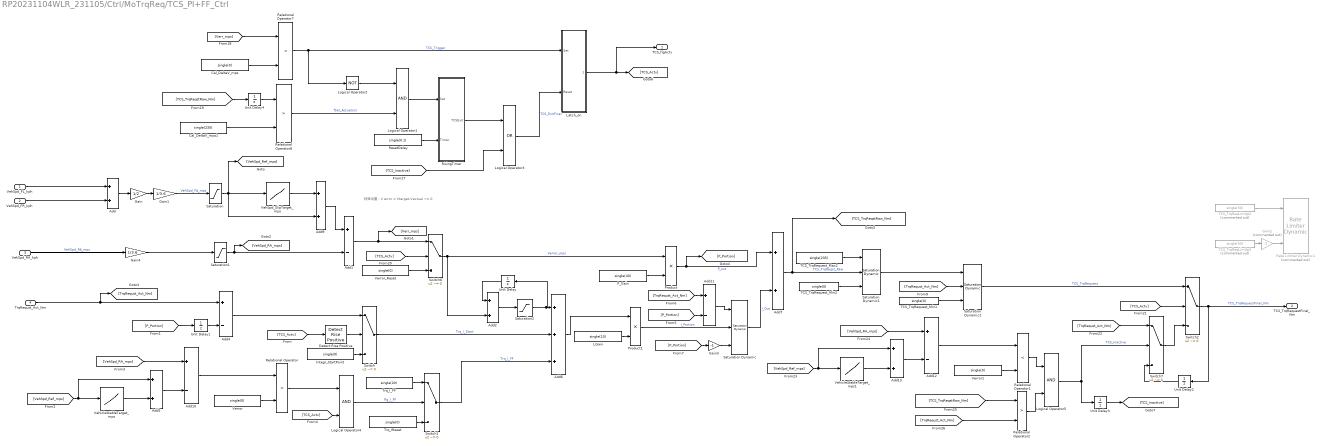
== system RP20231104WLR_231105/Ctrl/MoTrqReq/TCS_PI+FF_Ctrl ==
  note: 特殊设置：V error = Vtarget-Vactual <= 0
  VehSpd_FL_kph : Inport
  VehSpd_FR_kph : Inport  Port=2
  VehSpd_RA_kph : Inport  Port=3
  TrqRequst_Act_Nm : Inport  Port=4
  Add{,2,5,7,9,13} (6 alike) : Sum
  Add{1,4,10..12} (5 alike) : Sum  Inputs=+-
  Add6 : Sum  Inputs=+++
  Cal_DeltaV_mps : Constant  Value=single(0)
  Cal_DeltaV_mps1 : Constant  Value=single(235)
  Detect Rise Positive : simulink/Logic and Bit Operations/Detect Rise Positive  vinit=0  OutDataTypeStr=boolean
  Gain : Gain  Gain=1/2
  Gain1 : Gain  Gain=1/3.6
  Gain2 : Gain  Commented=on  Gain=-1
  Gain3 : Gain  Gain=-1
  Gain4 : Gain  Gain=1/3.6
  I_Gain : Constant  Value=single(10)
  Integr_StartPoint : Constant  Value=single(0)
  Latch_on : Subsystem
  Logical Operator1 : Logic  AllPortsSameDT=off  OutDataTypeStr=boolean
  Logical Operator2 : Logic  Operator=NOT  AllPortsSameDT=off  OutDataTypeStr=boolean
  Logical Operator3 : Logic  Operator=OR  AllPortsSameDT=off  OutDataTypeStr=boolean
  Logical Operator4 : Logic  AllPortsSameDT=off  OutDataTypeStr=boolean
  Logical Operator5 : Logic  AllPortsSameDT=off  OutDataTypeStr=boolean
  P_Gain : Constant  Value=single(40)
  Product : Product
  Product1 : Product
  Rate Limiter Dynamic1 : simulink/Discontinuities/Rate Limiter Dynamic  Commented=on
  Relational Operator : RelationalOperator  Operator=<  OutDataTypeStr=boolean  RndMeth=Simplest
  Relational Operator1 : RelationalOperator  Operator=<  OutDataTypeStr=boolean  RndMeth=Simplest
  Relational Operator2 : RelationalOperator  Operator=>  OutDataTypeStr=boolean  RndMeth=Simplest
  Relational Operator7 : RelationalOperator  Operator=<  OutDataTypeStr=boolean  RndMeth=Simplest
  Relational Operator8 : RelationalOperator  Operator=>  OutDataTypeStr=boolean  RndMeth=Simplest
  ResetDelay : Constant  Value=single(0.1)
  RisingTimer : Subsystem
  Saturation : Saturate  UpperLimit=40  LowerLimit=0
  Saturation Dynamic : simulink/Discontinuities/Saturation Dynamic  OutMin=[]  OutMax=[]  OutDataTypeStr=Inherit: Same as second input  OutDataType=fixdt(1, 16)  OutScaling=2^-10  DoSatur=off
  Saturation Dynamic1 : simulink/Discontinuities/Saturation Dynamic  OutMin=[]  OutMax=[]  OutDataTypeStr=Inherit: Same as second input  OutDataType=fixdt(1, 16)  OutScaling=2^-10  DoSatur=off
  Saturation Dynamic2 : simulink/Discontinuities/Saturation Dynamic  OutMin=[]  OutMax=[]  OutDataTypeStr=Inherit: Same as second input  OutDataType=fixdt(1, 16)  OutScaling=2^-10  DoSatur=off
  Saturation1 : Saturate  UpperLimit=50  LowerLimit=0
  Saturation2 : Saturate  UpperLimit=400  LowerLimit=-100
  Switch{,1..2,6..7} (5 alike) : Switch  Criteria=u2 ~= 0
  TCS_TrqReqLimUp2 : Constant  Commented=on  Value=single(50)
  TCS_TrqReqLimUp3 : Constant  Commented=on  Value=single(50)
  TCS_TrqRequest_Max2 : Constant  Value=single(235)
  TCS_TrqRequest_Min1 : Constant  Value=single(0)
  TCS_TrqRequest_Min2 : Constant  Value=single(0)
  Trq_IReset : Constant  Value=single(0)
  Trq_I_FF : Constant  Value=single(20)
  Unit Delay{,1..4} (5 alike) : UnitDelay  SampleTime=-1
  VehSpd_SlipTarget_mps : Lookup_n-D  NumberOfTableDimensions=1  BreakpointsForDimension1=[0,3,25,30]  Table=[0.3,0.3,2.5,2.5]  ExtrapMethod=Clip  InternalRulePriority=Speed  RndMeth=Simplest  InputSameDT=on
  VehicleStableTarget_mps : Lookup_n-D  NumberOfTableDimensions=1  BreakpointsForDimension1=[0,3,25,30]  Table=[0.4,0.4,1.2,1.2]  ExtrapMethod=Clip  InternalRulePriority=Speed  RndMeth=Simplest  InputSameDT=on
  VehicleStableTarget_mps1 : Lookup_n-D  NumberOfTableDimensions=1  BreakpointsForDimension1=[0,3,25,30]  Table=[0.4,0.4,1.2,1.2]  ExtrapMethod=Clip  InternalRulePriority=Speed  RndMeth=Simplest  InputSameDT=on
  Verror : Constant  Value=single(0)
  Verror1 : Constant  Value=single(0)
  Verror_Reset : Constant  Value=single(0)
  TCS_flgActv : Outport  VectorParamsAs1DForOutWhenUnconnected=on
  TCS_TrqRequestFinal_Nm : Outport  Port=2  VectorParamsAs1DForOutWhenUnconnected=on
  wires:
  Add1/1 -> Switch6/1, [Verr_mps]
  Switch2/1 -> TCS_TrqRequestFinal_Nm/1, Unit Delay2/1  "TCS_TrqRequestFinal_Nm"
  Saturation/1 -> Add9/2, VehSpd_SlipTarget_mps/1, [VehSpd_Ref_mps]
  Gain3/1 -> Saturation Dynamic/3
  [P_Portion] -> Gain3/1
  P_Gain/1 -> Product/2
  Unit Delay/1 -> Add2/1
  Add2/1 -> Saturation2/1
  [TrqRequst_Act_Nm] -> Add11/1
  Saturation2/1 -> Unit Delay/1, Add6/1
  Switch/1 -> Add6/2  "Trq_I_Start"
  Saturation Dynamic/1 -> Add7/2  "I_Out"
  Gain1/1 -> Saturation/1  "VehSpd_FA_mps"
  Saturation1/1 -> Add1/2, [VehSpd_RA_mps]
  Product1/1 -> Saturation Dynamic/2  "I_Portion"
  TrqRequst_Act_Nm/1 -> Add4/1, [TrqRequst_Act_Nm]
  Add6/1 -> Product1/1
  TCS_TrqRequest_Min1/1 -> Saturation Dynamic2/3
  Add/1 -> Gain/1
  Gain/1 -> Gain1/1
  Detect Rise Positive/1 -> Switch/2
  Integr_StartPoint/1 -> Switch/3
  I_Gain/1 -> Product1/2
  Saturation Dynamic2/1 -> Switch2/1  "TCS_TrqRequest"
  Add7/1 -> Saturation Dynamic1/2, [TCS_TrqReqstRaw_Nm]  "TCS_TrqReqst_Raw"
  [TrqRequst_Act_Nm] -> Saturation Dynamic2/2
  VehSpd_FL_kph/1 -> Add/1
  VehSpd_RA_kph/1 -> Gain4/1
  VehSpd_FR_kph/1 -> Add/2
  VehSpd_SlipTarget_mps/1 -> Add9/1
  Add9/1 -> Add1/1
  [Verr_mps] -> Relational Operator7/1
  Cal_DeltaV_mps/1 -> Relational Operator7/2
  Relational Operator7/1 -> Latch_on/1(Set), Logical Operator2/1  "TCS_Trigger"
  [TCS_TrqReqstRaw_Nm] -> Unit Delay4/1
  Logical Operator2/1 -> Logical Operator1/1
  Relational Operator8/1 -> Logical Operator1/2  "fSat_Actuators"
  Cal_DeltaV_mps1/1 -> Relational Operator8/2
  Logical Operator1/1 -> RisingTimer/1(Set)
  ResetDelay/1 -> RisingTimer/2(Timer)
  RisingTimer/1(TCSExit) -> Logical Operator3/1
  Logical Operator3/1 -> Latch_on/2(Reset)  "TCS_ExitFinal"
  Latch_on/1(flg_TCSActv) -> TCS_flgActv/1, [TCS_Actv]
  [TCS_Actv] -> Switch6/2
  Verror_Reset/1 -> Switch6/3
  Switch6/1 -> Product/1, Add2/2  "Verror_mps"
  Product/1 -> [P_Portion], Add7/1  "P_out"
  [TCS_Actv] -> Detect Rise Positive/1
  [P_Portion] -> Unit Delay1/1
  Add4/1 -> Switch/1
  Unit Delay1/1 -> Add4/2
  [VehSpd_Ref_mps] -> Add5/1, VehicleStableTarget_mps/1
  VehicleStableTarget_mps/1 -> Add5/2
  Add5/1 -> Add10/2
  [VehSpd_RA_mps] -> Add10/1
  Add10/1 -> Relational Operator/1
  Verror/1 -> Relational Operator/2
  Relational Operator/1 -> Logical Operator4/1
  [TCS_Actv] -> Logical Operator4/2
  Logical Operator4/1 -> Switch1/2  "flg_I_FF"
  Trq_I_FF/1 -> Switch1/1
  Trq_IReset/1 -> Switch1/3
  Switch1/1 -> Add6/3  "Trq_I_FF"
  [P_Portion] -> Add11/2
  Add11/1 -> Saturation Dynamic/1
  [TCS_Actv] -> Switch2/2
  Switch7/1 -> Switch2/3
  [TrqRequst_Act_Nm] -> Switch7/1
  Verror1/1 -> Relational Operator1/2
  Add12/1 -> Relational Operator1/1
  [VehSpd_RA_mps] -> Add12/1
  Add13/1 -> Add12/2
  VehicleStableTarget_mps1/1 -> Add13/2
  [VehSpd_Ref_mps] -> VehicleStableTarget_mps1/1, Add13/1
  [TCS_TrqReqstRaw_Nm] -> Relational Operator2/1
  [TrqRequst_Act_Nm] -> Relational Operator2/2
  Relational Operator1/1 -> Logical Operator5/1
  Relational Operator2/1 -> Logical Operator5/2
  Logical Operator5/1 -> Unit Delay3/1, Switch7/2  "TCS_Inactive"
  Unit Delay2/1 -> Switch7/3
  Unit Delay3/1 -> [TCS_Inactive]
  [TCS_Inactive] -> Logical Operator3/2
  Unit Delay4/1 -> Relational Operator8/1
  TCS_TrqReqLimUp2/1 -> Rate Limiter Dynamic1/1
  Gain2/1 -> Rate Limiter Dynamic1/3
  TCS_TrqReqLimUp3/1 -> Gain2/1
  Gain4/1 -> Saturation1/1  "VehSpd_RA_mps"
  Saturation Dynamic1/1 -> Saturation Dynamic2/1
  TCS_TrqRequest_Max2/1 -> Saturation Dynamic1/1
  TCS_TrqRequest_Min2/1 -> Saturation Dynamic1/3

== system RP20231104WLR_231105/Input/MCU_RECIEVE/MCU_pwr ==
  CANOK : Inport
  ID : Inport  Port=2
  Msg : Inport  Port=3
  function : TriggerPort  TriggerType=function-call  VariantControl=(inherit)
  Bus Creator3 : BusCreator  Inputs=6
  MCU_VCUMeter1 : Subsystem  TreatAsAtomicUnit=on
  MCU_pwr : Outport  VectorParamsAs1DForOutWhenUnconnected=on
  wires:
  Bus Creator3/1 -> MCU_pwr/1
  Msg/1 -> MCU_VCUMeter1/2(Msg)
  CANOK/1 -> MCU_VCUMeter1/Enable
  ID/1 -> MCU_VCUMeter1/1(ID)
  MCU_VCUMeter1/1("AC_current ") -> Bus Creator3/1  "AC_current"
  MCU_VCUMeter1/2(MCU_temp) -> Bus Creator3/2  "MCU_temp"
  MCU_VCUMeter1/3(current) -> Bus Creator3/3  "current"
  MCU_VCUMeter1/4(motor_temp) -> Bus Creator3/4  "motor_temp"
  MCU_VCUMeter1/5(voltage) -> Bus Creator3/5  "voltage"
  MCU_VCUMeter1/6(power) -> Bus Creator3/6  "power"

== system RP20231104WLR_231105/Input/MCU_RECIEVE/MCU_state ==
  CANOK : Inport
  ID : Inport  Port=2
  Msg : Inport  Port=3
  function : TriggerPort  TriggerType=function-call  VariantControl=(inherit)
  Bus Creator3 : BusCreator  Inputs=16
  MCU_state : Subsystem  TreatAsAtomicUnit=on
  Out1 : Outport
  wires:
  Msg/1 -> MCU_state/2(Msg)
  CANOK/1 -> MCU_state/Enable
  ID/1 -> MCU_state/1(ID)
  Bus Creator3/1 -> Out1/1
  MCU_state/1(12V_error) -> Bus Creator3/1
  MCU_state/2(alarm) -> Bus Creator3/2
  MCU_state/3(undervol) -> Bus Creator3/3
  MCU_state/4(controller_ready) -> Bus Creator3/4
  MCU_state/5(MCU_temp_warn) -> Bus Creator3/5
  MCU_state/6(mode_cmd8) -> Bus Creator3/6
  MCU_state/7(motor_temp_warn) -> Bus Creator3/7
  MCU_state/8(overcur) -> Bus Creator3/8
  MCU_state/9(pow_lim_warn) -> Bus Creator3/9
  MCU_state/10(overvol) -> Bus Creator3/10
  MCU_state/11(precharge) -> Bus Creator3/11
  MCU_state/12(rotation_warn) -> Bus Creator3/12
  MCU_state/13(selfcech) -> Bus Creator3/13
  MCU_state/14(RPM) -> Bus Creator3/14
  MCU_state/15(torque) -> Bus Creator3/15
  MCU_state/16(Spd_R) -> Bus Creator3/16  "Spd_R_kph"

== system RP20231104WLR_231105/Ctrl/MoTrqReq/TCS_PI+FF_Ctrl/Latch_on ==
  Set : Inport
  Reset : Inport  Port=2
  Logical Operator4 : Logic  Operator=NOR  AllPortsSameDT=off  OutDataTypeStr=boolean
  Logical Operator5 : Logic  Operator=NOR  AllPortsSameDT=off  OutDataTypeStr=boolean
  Unit Delay1 : UnitDelay  SampleTime=-1
  flg_TCSActv : Outport  VectorParamsAs1DForOutWhenUnconnected=on
  wires:
  Logical Operator5/1 -> flg_TCSActv/1, Unit Delay1/1
  Reset/1 -> Logical Operator5/2
  Unit Delay1/1 -> Logical Operator4/1
  Set/1 -> Logical Operator4/2
  Logical Operator4/1 -> Logical Operator5/1

== system RP20231104WLR_231105/Ctrl/MoTrqReq/TCS_PI+FF_Ctrl/RisingTimer ==
  Set : Inport
  Timer : Inport  Port=2
  Add10 : Sum
  Min : MinMax  Inputs=2
  Relational Operator9 : RelationalOperator  OutDataTypeStr=boolean  RndMeth=Simplest
  Reset : Constant  Value=single(0)
  Steptime : Constant  Value=single(0.01)
  Switch6 : Switch  Criteria=u2 ~= 0
  Unit Delay1 : UnitDelay  SampleTime=-1
  TCSExit : Outport  VectorParamsAs1DForOutWhenUnconnected=on
  wires:
  Add10/1 -> Switch6/1
  Set/1 -> Switch6/2
  Min/1 -> Unit Delay1/1, Relational Operator9/1
  Unit Delay1/1 -> Add10/1
  Timer/1 -> Relational Operator9/2, Min/2
  Reset/1 -> Switch6/3
  Relational Operator9/1 -> TCSExit/1
  Steptime/1 -> Add10/2
  Switch6/1 -> Min/1
